simulink model "cart_pend"  (R2019a)
settings: Solver=FixedStepAuto  StartTime=0.0  StopTime=19.999  FixedStep=0.001  RelTol=1e-3
values from neighbouring files (symbols this model uses):
  h = 0.1    [finite_time_DP.m]    (also in prepare_sim.m = params.h)
  X0 = [0; 0; pi/6; 0]    [prepare_sim.m]
undefined symbols (not defined in the file or in its folder): finite_time_DP, x0, xf
settings Model: Creator=Piku  LastModifiedBy=Piku

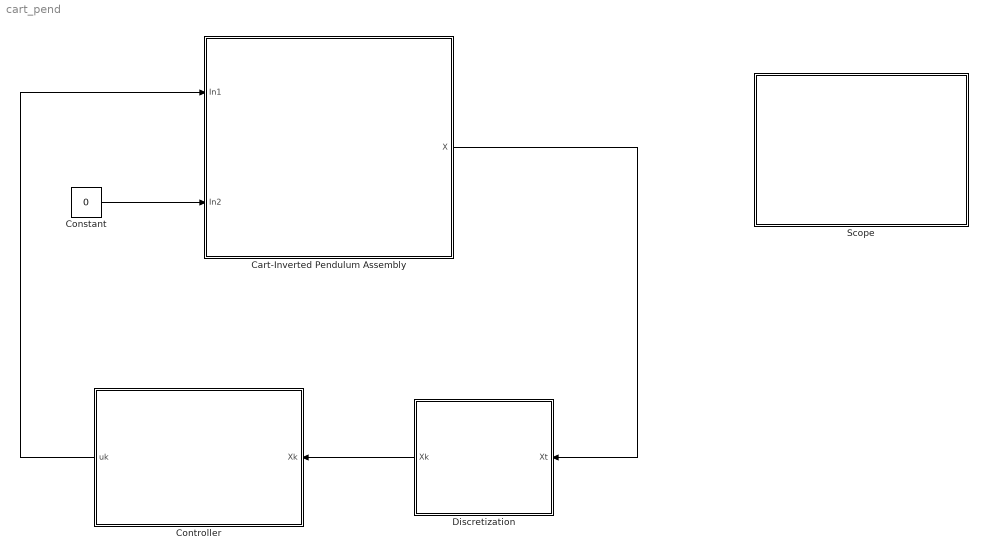
== system cart_pend ==
  Cart-Inverted Pendulum Assembly : Subsystem
      mask Display: image('cart_pendulum.png');
  Constant : Constant  Value=0
  Controller : Subsystem
  Discretization : Subsystem
  Scope : Subsystem
  wires:
  Cart-Inverted Pendulum Assembly/1("X ") -> Discretization/1(Xt)
  Controller/1(uk) -> Cart-Inverted Pendulum Assembly/1(In1)
  Constant/1 -> Cart-Inverted Pendulum Assembly/2(In2)
  Discretization/1(Xk) -> Controller/1(" Xk")

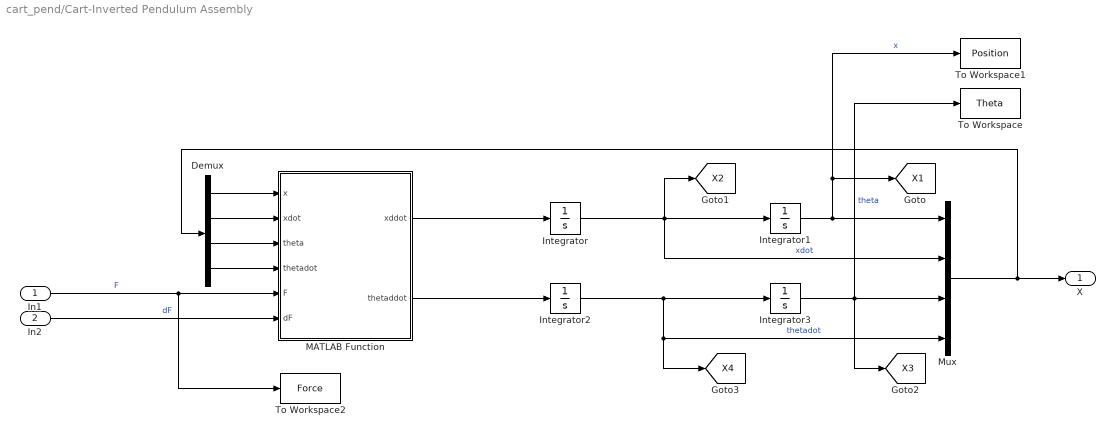
== system cart_pend/Cart-Inverted Pendulum Assembly ==
  In1 : Inport  PortDimensions=1
  In2 : Inport  Port=2  PortDimensions=1
  Demux : Demux
  Integrator : Integrator  InitialCondition=X0(2)  LimitOutput=on  UpperSaturationLimit=1e6  LowerSaturationLimit=-1e6
  Integrator1 : Integrator  InitialCondition=X0(1)  UpperSaturationLimit=xf  LowerSaturationLimit=-x0
  Integrator2 : Integrator  InitialCondition=X0(4)  LimitOutput=on  UpperSaturationLimit=1e6  LowerSaturationLimit=-1e6
  Integrator3 : Integrator  InitialCondition=X0(3)  LimitOutput=on  UpperSaturationLimit=pi  LowerSaturationLimit=-pi
  MATLAB Function : MATLAB Function  TreatAsAtomicUnit=on
  Mux : Mux
  To Workspace : ToWorkspace  VariableName=Theta  SaveFormat=Timeseries  SampleTime=-1
  To Workspace1 : ToWorkspace  VariableName=Position  SaveFormat=Timeseries  SampleTime=-1
  To Workspace2 : ToWorkspace  VariableName=Force  SaveFormat=Timeseries  SampleTime=-1
  "X " : Outport  PortDimensions=4
  tag scope: X1=global, X2=global, X3=global, X4=global
  wires:
  Integrator2/1 -> Integrator3/1, [X4], Mux/4  "thetadot"
  In1/1 -> To Workspace2/1, MATLAB Function/5(F)  "F"
  Integrator3/1 -> [X3], To Workspace/1, Mux/3  "theta"
  Integrator/1 -> [X2], Mux/2, Integrator1/1  "xdot"
  Integrator1/1 -> [X1], To Workspace1/1, Mux/1  "x"
  Mux/1 -> Demux/1, "X "/1
  MATLAB Function/1(xddot) -> Integrator/1
  MATLAB Function/2(thetaddot) -> Integrator2/1
  Demux/1 -> MATLAB Function/1(x)
  Demux/2 -> MATLAB Function/2(xdot)
  Demux/3 -> MATLAB Function/3(theta)
  Demux/4 -> MATLAB Function/4(thetadot)
  In2/1 -> MATLAB Function/6(dF)  "dF"

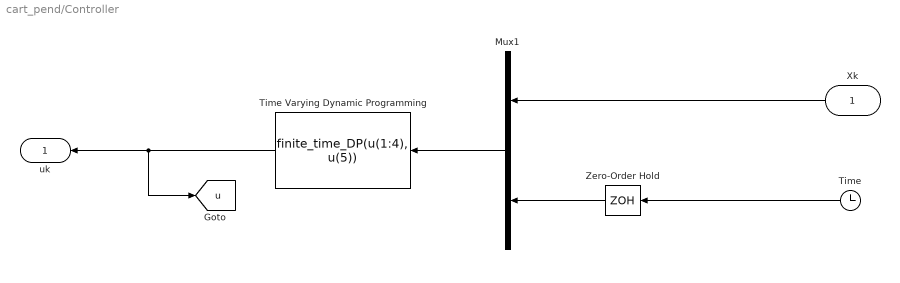
== system cart_pend/Controller ==
  " Xk" : Inport  PortDimensions=4
  Mux1 : Mux  Inputs=2
  Time : Clock
  Time Varying Dynamic Programming : MATLABFcn  MATLABFcn=finite_time_DP(u(1:4), u(5))  OutputDimensions=1
  Zero-Order Hold : ZeroOrderHold  SampleTime=-1
  uk : Outport
  tag scope: u=global
  wires:
  Zero-Order Hold/1 -> Mux1/2
  Time/1 -> Zero-Order Hold/1
  Time Varying Dynamic Programming/1 -> [u], uk/1
  Mux1/1 -> Time Varying Dynamic Programming/1
  " Xk"/1 -> Mux1/1

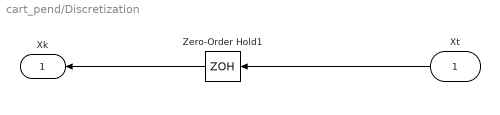
== system cart_pend/Discretization ==
  Xt : Inport
  Zero-Order Hold1 : ZeroOrderHold  SampleTime=h
  Xk : Outport
  wires:
  Zero-Order Hold1/1 -> Xk/1
  Xt/1 -> Zero-Order Hold1/1

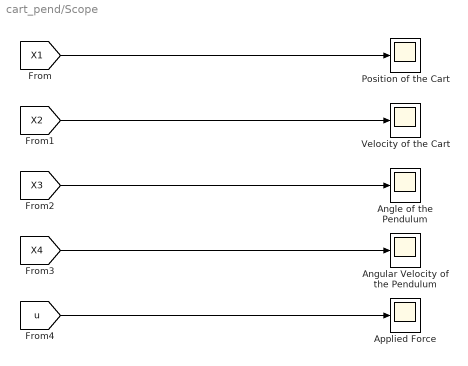
== system cart_pend/Scope ==
  Angle of the Pendulum : Scope
  Angular Velocity of the Pendulum : Scope
  Applied Force : Scope
  Position of the Cart : Scope
  Velocity of the Cart : Scope
  wires:
  [X1] -> Position of the Cart/1
  [X2] -> Velocity of the Cart/1
  [X3] -> Angle of the Pendulum/1
  [X4] -> Angular Velocity of the Pendulum/1
  [u] -> Applied Force/1

== matlab function cart_pend/Cart-Inverted Pendulum Assembly/MATLAB Function ==
  data: x input; xddot output; xdot input; theta input; thetadot input; F input; thetaddot output; dF input
function [xddot, thetaddot] = fcn(x, xdot, theta, thetadot, F, dF)

M   = 0.5;          % Mass of the cart      
m   = 0.2;          % Mass of the inverted pendulum
bc  = 0.1;          % coefficient of friction for cart
l   = 0.3;          % length to the pendulum center of mass
I   = 0.006;        % moment of inertia of the pendulum
bp  = 0.012;        % coefficient of friction for pendulum
g   = 9.8;          % acceleration due to gravity

% Dynamics of the pendulum
ap0 = (I + m*l^2);
ap1 = -(m^2*l^2)/(M+m);
bp0 = (m*l)/(M+m);
bp1 = 0.5*(m^2*l^2)/(M+m);
bp2 = (m*l*bc)/(M+m);
bp3 = bp;
bp4 = -m*g*l; 
bp5 = -l;
thetaddot = (1/(ap0 + ap1*cos(theta)^2))* ( bp0*cos(theta)*(F - dF) ...
             - bp1*thetadot^2*sin(2*theta) - bp2*cos(theta)*xdot ...
             - bp3*thetadot - bp4*sin(theta) - bp5*cos(theta)*dF );

% Dynamics of the cart
ac0 = M + m;
ac1 = - m^2*l^2/(I + m*l^2);
bc0 = 1;
bc1 = m*l;
bc2 = bc;
bc3 = (bp*m*l)/(I + m*l^2);
bc4 = -0.5*(m^2*l^2*g)/(I + m*l^2);
bc5 = -(m*l^2)/(I + m*l^2);
xddot = (1/(ac0 + ac1*cos(theta)^2))* (bc0*(F - dF)...
             - bc1*thetadot^2*sin(theta) - bc2*xdot ...
             - bc3*thetadot*cos(theta) - bc4*sin(2*theta) ...
             - bc5*dF*cos(theta)^2 );
end
